simulink model "six_plus_six_AcmsteeringV10_main"  (R2014a)
settings: Solver=FixedStepDiscrete  StartTime=0.0  StopTime=10.0  FixedStep=0.0005  RelTol=1e-3
InitFcn:
  | Veh_Par_wxt
values from neighbouring files (symbols this model uses):
  acc_spdctl = [0 100]    [Veh_Par_wxt.m]
  ag_thr = ecucoder_cal(ag_thr)    [Veh_Par_wxt.m]
  B = 1.8    [Veh_Par_wxt.m]
  bra_em = 100    [Veh_Par_wxt.m]
  bra_pre_gz2 = 100/3    (= 33.3333333333)    [Veh_Par_wxt.m]
  bra_pre_gz34 = 10/3    (= 3.33333333333)    [Veh_Par_wxt.m]
  bra_pre_yd = 10/2    (= 5)    [Veh_Par_wxt.m]
  brakepre_dem_data = [0 1 2 3 4 5 6 7 8 9 10]    [Veh_Par_wxt.m]
  brakeTrq_dem_data = [0 125 251 376 502 627 753 878 1004 1129 1255]    [Veh_Par_wxt.m]
  bratrq_max = 4*1255    (= 5020)    [Veh_Par_wxt.m]
  eff_tran = 0.9    [Veh_Par_wxt.m]
  ESP_switch = ecucoder_cal(ESP_switch)    [Veh_Par_wxt.m]
  G = Mass*g    (= 15696)    [Veh_Par_wxt.m]
  kd1 = ecucoder_cal(kd1)    [Veh_Par_wxt.m]
  kd2 = 0    [Veh_Par_wxt.m]
  ki1 = ecucoder_cal(ki1)    [Veh_Par_wxt.m]
  ki2 = 1    [Veh_Par_wxt.m]
  kp1 = ecucoder_cal(kp1)    [Veh_Par_wxt.m]
  kp2 = 300    [Veh_Par_wxt.m]
  L = L1+L2    (= 2.9)    [Veh_Par_wxt.m]
  premax = 100    [Veh_Par_wxt.m]
  Radius = 0.4572/2    (= 0.2286)    [Veh_Par_wxt.m]
  RC_switch = ecucoder_cal(RC_switch)    [Veh_Par_wxt.m]
  s_opt_yi = 0.15    [Veh_Par_wxt.m]
  s_opt_zhuan = 0.8    [Veh_Par_wxt.m]
  s_opt_zhuan_add = 0.05    [Veh_Par_wxt.m]
  s_opt_zhuan_table = [0.8 0.8 0.3 0.3]    [Veh_Par_wxt.m]
  spd_map_mot = [0 499.85 999.79 1500 2000 2500 3000 3500 4000 4500 4999.8 5999.8]    [Veh_Par_wxt.m]
  spd_spdctl = [0 500]    [Veh_Par_wxt.m]
  speed_thr_park = 5/3.6/Radius*tras_ratio*30/pi    (= 464.143899364)    [Veh_Par_wxt.m]
  TCS_switch = ecucoder_cal(TCS_switch)    [Veh_Par_wxt.m]
  tras_ratio = 8    [Veh_Par_wxt.m]
  trq_map_mot = [70.5 70.012 71.154 65.797 53.917 45.159 38.073 32.685 27.48 17.133 14.949 10.07]    [Veh_Par_wxt.m]
  trqmax_yd = 70.5    [Veh_Par_wxt.m]
  trqmax_zx = 70.5    [Veh_Par_wxt.m]
  trqmaxneg = -70.5    [Veh_Par_wxt.m]
  v_gain = 0.9    [Veh_Par_wxt.m]
  v_table = [0 5 20 100]    [Veh_Par_wxt.m]
  v_thr_park = 5    [Veh_Par_wxt.m]
  zhidong_bianmazhi = [-140000 750000]    [Veh_Par_wxt.m]
  zhidong_down = -140000    [Veh_Par_wxt.m]
  zhidong_up = 750000    [Veh_Par_wxt.m]
  zhidong_youmen = [0 100]    [Veh_Par_wxt.m]
  zhuanxiang_bianmazhi = [-400000 0 400000]    [Veh_Par_wxt.m]
  zhuanxiang_down = -400000    [Veh_Par_wxt.m]
  zhuanxiang_up = 400000    [Veh_Par_wxt.m]
  zhuanxiang_youmen = [-100 0 100]    [Veh_Par_wxt.m]
undefined symbols (not defined in the file or in its folder): ecucoder_acal, guzhang_lf, guzhang_lm, guzhang_lr, guzhang_rf, guzhang_rm, guzhang_rr, myFIS
libraries: simulink x979, ec5744lib x59, fuzblock x2
(part 5 of 27)

== system six_plus_six_AcmsteeringV10_main/Data_input/2/Enabled Subsystem ==
  In2 : Inport
  Enable : EnablePort
  Add : Sum
  Constant : Constant  Value=256
  Constant1 : Constant  SampleTime=-1
  Constant3 : Constant  Value=256
  Data Type Conversion{8..13} (6 alike) : DataTypeConversion  OutDataTypeStr=uint8
  Demux1 : Demux  Outputs=6
  MATLAB Function1 : MATLAB Function  TreatAsAtomicUnit=on
  MATLAB Function3 : MATLAB Function  TreatAsAtomicUnit=on
  Memory : Memory  InheritSampleTime=on
  Product : Product
  Product2 : Product
  Saturation : Saturate  UpperLimit=5  LowerLimit=0
  Sum : Sum  Inputs=|++
  Sum1 : Sum  Inputs=|++
  Terminator1 : Terminator
  Terminator2 : Terminator
  motec_spd_4 : Outport
  motec_current_4 : Outport  Port=2
  enable_count1 : Outport  Port=3
  wires:
  MATLAB Function1/1(current_out) -> motec_current_4/1
  MATLAB Function3/1(speed_out) -> motec_spd_4/1
  Sum1/1 -> MATLAB Function1/1(current_in)
  Data Type Conversion13/1 -> Sum1/1
  Product2/1 -> Sum1/2
  Constant3/1 -> Product2/1
  Data Type Conversion12/1 -> Product2/2
  Sum/1 -> MATLAB Function3/1(speed)
  Product/1 -> Sum/2
  Constant/1 -> Product/1
  Data Type Conversion11/1 -> Product/2
  Data Type Conversion10/1 -> Sum/1
  Data Type Conversion9/1 -> Terminator2/1
  Data Type Conversion8/1 -> Terminator1/1
  Demux1/6 -> Data Type Conversion12/1
  Demux1/5 -> Data Type Conversion13/1
  Demux1/4 -> Data Type Conversion11/1
  Demux1/3 -> Data Type Conversion10/1
  Demux1/2 -> Data Type Conversion9/1
  Demux1/1 -> Data Type Conversion8/1
  In2/1 -> Demux1/1
  Constant1/1 -> Add/1
  Memory/1 -> Add/2
  Add/1 -> Saturation/1
  Saturation/1 -> enable_count1/1, Memory/1

== system six_plus_six_AcmsteeringV10_main/Data_input/3/Enabled Subsystem ==
  In2 : Inport
  Enable : EnablePort
  Add : Sum
  Constant : Constant  Value=256
  Constant1 : Constant  SampleTime=-1
  Constant3 : Constant  Value=256
  Data Type Conversion{8..13} (6 alike) : DataTypeConversion  OutDataTypeStr=uint8
  Demux1 : Demux  Outputs=6
  MATLAB Function1 : MATLAB Function  TreatAsAtomicUnit=on
  MATLAB Function3 : MATLAB Function  TreatAsAtomicUnit=on
  Memory : Memory  InheritSampleTime=on
  Product : Product
  Product2 : Product
  Saturation : Saturate  UpperLimit=5  LowerLimit=0
  Sum : Sum  Inputs=|++
  Sum1 : Sum  Inputs=|++
  Terminator1 : Terminator
  Terminator2 : Terminator
  motec_spd_3 : Outport
  motec_current_3 : Outport  Port=2
  enable_count1 : Outport  Port=3
  wires:
  MATLAB Function1/1(current_out) -> motec_current_3/1
  MATLAB Function3/1(speed_out) -> motec_spd_3/1
  Sum1/1 -> MATLAB Function1/1(current_in)
  Data Type Conversion13/1 -> Sum1/1
  Product2/1 -> Sum1/2
  Constant3/1 -> Product2/1
  Data Type Conversion12/1 -> Product2/2
  Sum/1 -> MATLAB Function3/1(speed)
  Product/1 -> Sum/2
  Constant/1 -> Product/1
  Data Type Conversion11/1 -> Product/2
  Data Type Conversion10/1 -> Sum/1
  Data Type Conversion9/1 -> Terminator2/1
  Data Type Conversion8/1 -> Terminator1/1
  Demux1/6 -> Data Type Conversion12/1
  Demux1/5 -> Data Type Conversion13/1
  Demux1/4 -> Data Type Conversion11/1
  Demux1/3 -> Data Type Conversion10/1
  Demux1/2 -> Data Type Conversion9/1
  Demux1/1 -> Data Type Conversion8/1
  In2/1 -> Demux1/1
  Constant1/1 -> Add/1
  Memory/1 -> Add/2
  Add/1 -> Saturation/1
  Saturation/1 -> enable_count1/1, Memory/1

== system six_plus_six_AcmsteeringV10_main/Data_input/4/Enabled Subsystem ==
  In2 : Inport
  Enable : EnablePort
  Data Type Conversion{,1..7} (8 alike) : DataTypeConversion
  Demux1 : Demux  Outputs=8
  MATLAB Function : MATLAB Function  TreatAsAtomicUnit=on
  MATLAB Function1 : MATLAB Function  TreatAsAtomicUnit=on
  Xangularrate_Out : Outport
  Yangularrate_Out : Outport  Port=2
  wires:
  In2/1 -> Demux1/1
  Demux1/4 -> Data Type Conversion3/1
  Demux1/3 -> Data Type Conversion2/1
  Demux1/2 -> Data Type Conversion1/1
  Demux1/1 -> Data Type Conversion/1
  MATLAB Function/1(y) -> Xangularrate_Out/1
  MATLAB Function1/1(y) -> Yangularrate_Out/1
  Demux1/5 -> Data Type Conversion4/1
  Demux1/6 -> Data Type Conversion5/1
  Demux1/7 -> Data Type Conversion6/1
  Demux1/8 -> Data Type Conversion7/1
  Data Type Conversion/1 -> MATLAB Function/1(data1)
  Data Type Conversion1/1 -> MATLAB Function/2(data2)
  Data Type Conversion2/1 -> MATLAB Function/3(data3)
  Data Type Conversion3/1 -> MATLAB Function/4(data4)
  Data Type Conversion4/1 -> MATLAB Function1/1(data1)
  Data Type Conversion5/1 -> MATLAB Function1/2(data2)
  Data Type Conversion6/1 -> MATLAB Function1/3(data3)
  Data Type Conversion7/1 -> MATLAB Function1/4(data4)

== matlab function six_plus_six_AcmsteeringV10_main/MainControl/mode_control/center_steer/center_steer/容错控制/MATLAB Function ==
  data: trq_dem_l input; trq_dem_lf output; trq_dem_lm output; trq_dem_r input; trqlim_lf input; trqlim_lm input; trqlim_lr input; trqlim_rf input; trqlim_rm input; trqlim_rr input; guzhang_lf input; guzhang_lm input; guzhang_lr input; guzhang_rf input; guzhang_rm input; guzhang_rr input; trq_dem_lr output; trq_dem_rf output; trq_dem_rm output; trq_dem_rr output; bra_pre_l output; bra_pre_r output; bra_pre_yd input; mode output; bra_dem_l input; bra_dem_r input; brake_dem input
function [trq_dem_lf,trq_dem_lm,trq_dem_lr,trq_dem_rf,trq_dem_rm,trq_dem_rr,bra_pre_l,bra_pre_r,mode] = fcn(trq_dem_l,trq_dem_r,trqlim_lf,trqlim_lm,trqlim_lr,trqlim_rf,trqlim_rm,trqlim_rr,guzhang_lf,guzhang_lm,guzhang_lr,guzhang_rf,guzhang_rm,guzhang_rr,bra_pre_yd,bra_dem_l,bra_dem_r,brake_dem)
%#codegen
if brake_dem==0
    
    trq_dem_lf=single(trq_dem_l/3);
    trq_dem_lm=single(trq_dem_l/3);
    trq_dem_lr=single(trq_dem_l/3);
    trq_dem_rf=single(trq_dem_r/3);
    trq_dem_rm=single(trq_dem_r/3);
    trq_dem_rr=single(trq_dem_r/3);
    bra_pre_l=single(0);
    bra_pre_r=single(0);
    mode=1;
    
    
    %     if guzhang_lf==0 && guzhang_lr==0 && guzhang_rf==0 && guzhang_rr==0    %0电机故障,平均分配
    %         trq_dem_lf=single(trq_dem_l/2);
    %         trq_dem_lr=single(trq_dem_l/2);
    %         trq_dem_rf=single(trq_dem_r/2);
    %         trq_dem_rr=single(trq_dem_r/2);
    %         bra_pre_l=single(0);
    %         bra_pre_r=single(0);
    %         mode=1;
    %     elseif  guzhang_lf==1 && guzhang_lr==0 && guzhang_rf==0 && guzhang_rr==0  %1电机故障，同侧电机进行力矩转移,跟行车不同，对侧不降扭。
    %         trq_dem_lf=single(0);
    %         trq_dem_lr=single(min(trq_dem_l,trqlim_lr));
    %         trq_dem_rf=single(trq_dem_r/2);
    %         trq_dem_rr=single(trq_dem_r/2);
    %         bra_pre_l=single(0);
    %         bra_pre_r=single(0);
    %         mode=2;
    %     elseif  guzhang_lf==0 && guzhang_lr==1 && guzhang_rf==0 && guzhang_rr==0
    %         trq_dem_lf=single(min(trq_dem_l,trqlim_lf));
    %         trq_dem_lr=single(0);
    %         trq_dem_rf=single(trq_dem_r/2);
    %         trq_dem_rr=single(trq_dem_r/2);
    %         bra_pre_l=single(0);
    %         bra_pre_r=single(0);
    %         mode=3;
    %     elseif  guzhang_lf==0 && guzhang_lr==0 && guzhang_rf==1 && guzhang_rr==0
    %         trq_dem_rf=single(0);
    %         trq_dem_rr=single(min(trq_dem_r,trqlim_rr));
    %         trq_dem_lf=single(trq_dem_l/2);
    %         trq_dem_lr=single(trq_dem_l/2);
    %         bra_pre_l=single(0);
    %         bra_pre_r=single(0);
    %         mode=4;
    %     elseif  guzhang_lf==0 && guzhang_lr==0 && guzhang_rf==0 && guzhang_rr==1
    %         trq_dem_rf=single(min(trq_dem_r,trqlim_rf));
    %         trq_dem_rr=single(0);
    %         trq_dem_lf=single(trq_dem_l/2);
    %         trq_dem_lr=single(trq_dem_l/2);
    %         bra_pre_l=single(0);
    %         bra_pre_r=single(0);
    %         mode=5;
    %     elseif  guzhang_lf==1 && guzhang_lr==1 && guzhang_rf==0 && guzhang_rr==0  %2电机故障，左侧双电机故障，左侧履带施加制动，改为原地转向
    %         trq_dem_lf=single(0);
    %         trq_dem_lr=single(0);
    %         trq_dem_rf=single(trq_dem_r/2);
    %         trq_dem_rr=single(trq_dem_r/2);
    %         bra_pre_l=single(bra_pre_yd);
    %         bra_pre_r=single(0);
    %         mode=6;
    %     elseif  guzhang_lf==0 && guzhang_lr==0 && guzhang_rf==1 && guzhang_rr==1  %右侧双电机故障
    %         trq_dem_lf=single(trq_dem_l/2);
    %         trq_dem_lr=single(trq_dem_l/2);
    %         trq_dem_rf=single(0);
    %         trq_dem_rr=single(0);
    %         bra_pre_l=single(0);
    %         bra_pre_r=single(bra_pre_yd);
    %         mode=7;
    %     elseif  guzhang_lf==1 && guzhang_lr==0 && guzhang_rf==1 && guzhang_rr==0 %2电机故障，对侧双电机故障,有4种情况,前两电机故障
    %         trq_dem_lf=single(0);
    %         trq_dem_rf=single(0);
    %         trq_dem_lr=single(min(trq_dem_l,trqlim_lr));
    %         trq_dem_rr=single(min(trq_dem_r,trqlim_rr));
    %         bra_pre_l=single(0);
    %         bra_pre_r=single(0);
    %         mode=8;
    %     elseif  guzhang_lf==0 && guzhang_lr==1 && guzhang_rf==0 && guzhang_rr==1 %后两电机故障
    %         trq_dem_lr=single(0);
    %         trq_dem_rr=single(0);
    %         trq_dem_lf=single(min(trq_dem_l,trqlim_lf));
    %         trq_dem_rf=single(min(trq_dem_r,trqlim_rf));
    %         bra_pre_l=single(0);
    %         bra_pre_r=single(0);
    %         mode=9;
    %     elseif  guzhang_lf==1 && guzhang_lr==0 && guzhang_rf==0 && guzhang_rr==1 %左前电机和右后电机故障
    %         trq_dem_lf=single(0);
    %         trq_dem_rr=single(0);
    %         trq_dem_lr=single(min(trq_dem_l,trqlim_lr));
    %         trq_dem_rf=single(min(trq_dem_r,trqlim_rf));
    %         bra_pre_l=single(0);
    %         bra_pre_r=single(0);
    %         mode=10;
    %     elseif  guzhang_lf==0 && guzhang_lr==1 && guzhang_rf==1 && guzhang_rr==0 %左后电机和右前电机故障
    %         trq_dem_lr=single(0);
    %         trq_dem_rf=single(0);
    %         trq_dem_lf=single(min(trq_dem_l,trqlim_lf));
    %         trq_dem_rr=single(min(trq_dem_r,trqlim_rr));
    %         bra_pre_l=single(0);
    %         bra_pre_r=single(0);
    %         mode=11;
    %     elseif guzhang_lf==1 && guzhang_lr==1 && guzhang_rf==1 && guzhang_rr==0   % 三电机故障
    %         trq_dem_lf=single(0);
    %         trq_dem_lr=single(0);
    %         trq_dem_rf=single(0);
    %         trq_dem_rr=single(min(trq_dem_r,trqlim_rr));
    %         bra_pre_l=single(bra_pre_yd);
    %         bra_pre_r=single(0);
    %         mode=12;
    %     elseif guzhang_lf==1 && guzhang_lr==1 && guzhang_rf==0 && guzhang_rr==1
    %         trq_dem_lf=single(0);
    %         trq_dem_lr=single(0);
    %         trq_dem_rf=single(min(trq_dem_r,trqlim_rf));
    %         trq_dem_rr=single(0);
    %         bra_pre_l=single(bra_pre_yd);
    %         bra_pre_r=single(0);
    %         mode=13;
    %     elseif guzhang_lf==1 && guzhang_lr==0 && guzhang_rf==1 && guzhang_rr==1
    %         trq_dem_lf=single(0);
    %         trq_dem_lr=single(min(trq_dem_l,trqlim_lr));
    %         trq_dem_rf=single(0);
    %         trq_dem_rr=single(0);
    %         bra_pre_l=single(0);
    %         bra_pre_r=single(bra_pre_yd);
    %         mode=14;
    %     elseif guzhang_lf==0 && guzhang_lr==1 && guzhang_rf==1 && guzhang_rr==1
    %         trq_dem_lf=single(min(trq_dem_l,trqlim_lf));
    %         trq_dem_lr=single(0);
    %         trq_dem_rf=single(0);
    %         trq_dem_rr=single(0);
    %         bra_pre_l=single(0);
    %         bra_pre_r=single(bra_pre_yd);
    %         mode=15;
    %     else
    %         %     guzhang_lf==1 && guzhang_lr==1 && guzhang_rf==1 && guzhang_rr==1 %四电机故障
    %         trq_dem_lf=single(0);
    %         trq_dem_lr=single(0);
    %         trq_dem_rf=single(0);
    %         trq_dem_rr=single(0);
    %         bra_pre_l=single(0);
    %         bra_pre_r=single(0);
    %         mode=16;
    %     end
else
    trq_dem_lf=single(0);
    trq_dem_lm=single(0);
    trq_dem_lr=single(0);
    trq_dem_rf=single(0);
    trq_dem_rm=single(0);
    trq_dem_rr=single(0);
    bra_pre_l=single(bra_dem_l);
    bra_pre_r=single(bra_dem_r);
    mode=17;
end
trq_dem_lf=single(min(trqlim_lf,trq_dem_lf));trq_dem_lf=single(max(0,trq_dem_lf));
trq_dem_lm=single(min(trqlim_lm,trq_dem_lm));trq_dem_lm=single(max(0,trq_dem_lm));
trq_dem_lr=single(min(trqlim_lr,trq_dem_lr));trq_dem_lr=single(max(0,trq_dem_lr));
trq_dem_rf=single(min(trqlim_rf,trq_dem_rf));trq_dem_rf=single(max(0,trq_dem_rf));
trq_dem_rm=single(min(trqlim_rm,trq_dem_rm));trq_dem_rm=single(max(0,trq_dem_rm));
trq_dem_rr=single(min(trqlim_rr,trq_dem_rr));trq_dem_rr=single(max(0,trq_dem_rr));
bra_pre_l=single(bra_pre_l);
bra_pre_r=single(bra_pre_r);
end

== system six_plus_six_AcmsteeringV10_main/Data_input/5/Enabled Subsystem ==
  In2 : Inport
  Enable : EnablePort
  Data Type Conversion{,1..7} (8 alike) : DataTypeConversion
  Demux1 : Demux  Outputs=8
  MATLAB Function : MATLAB Function  TreatAsAtomicUnit=on
  MATLAB Function1 : MATLAB Function  TreatAsAtomicUnit=on
  Zangularrate_Out : Outport
  Xacceleration_Out : Outport  Port=2
  wires:
  Demux1/8 -> Data Type Conversion7/1
  Demux1/7 -> Data Type Conversion6/1
  Demux1/6 -> Data Type Conversion5/1
  Demux1/5 -> Data Type Conversion4/1
  MATLAB Function1/1(y) -> Xacceleration_Out/1
  MATLAB Function/1(y) -> Zangularrate_Out/1
  Demux1/1 -> Data Type Conversion/1
  Demux1/2 -> Data Type Conversion1/1
  Demux1/3 -> Data Type Conversion2/1
  Demux1/4 -> Data Type Conversion3/1
  In2/1 -> Demux1/1
  Data Type Conversion/1 -> MATLAB Function/1(data1)
  Data Type Conversion1/1 -> MATLAB Function/2(data2)
  Data Type Conversion2/1 -> MATLAB Function/3(data3)
  Data Type Conversion3/1 -> MATLAB Function/4(data4)
  Data Type Conversion4/1 -> MATLAB Function1/1(data1)
  Data Type Conversion5/1 -> MATLAB Function1/2(data2)
  Data Type Conversion7/1 -> MATLAB Function1/4(data4)
  Data Type Conversion6/1 -> MATLAB Function1/3(data3)

== system six_plus_six_AcmsteeringV10_main/Data_input/6/Enabled Subsystem ==
  In2 : Inport
  Enable : EnablePort
  Data Type Conversion{,1..7} (8 alike) : DataTypeConversion
  Demux1 : Demux  Outputs=8
  MATLAB Function : MATLAB Function  TreatAsAtomicUnit=on
  MATLAB Function1 : MATLAB Function  TreatAsAtomicUnit=on
  Yacceleration_Out : Outport
  Zacceleration_Out : Outport  Port=2
  wires:
  In2/1 -> Demux1/1
  Demux1/4 -> Data Type Conversion3/1
  Demux1/3 -> Data Type Conversion2/1
  Demux1/2 -> Data Type Conversion1/1
  Demux1/1 -> Data Type Conversion/1
  MATLAB Function/1(y) -> Yacceleration_Out/1
  MATLAB Function1/1(y) -> Zacceleration_Out/1
  Demux1/5 -> Data Type Conversion4/1
  Demux1/6 -> Data Type Conversion5/1
  Demux1/7 -> Data Type Conversion6/1
  Demux1/8 -> Data Type Conversion7/1
  Data Type Conversion7/1 -> MATLAB Function1/4(data4)
  Data Type Conversion2/1 -> MATLAB Function/3(data3)
  Data Type Conversion/1 -> MATLAB Function/1(data1)
  Data Type Conversion1/1 -> MATLAB Function/2(data2)
  Data Type Conversion4/1 -> MATLAB Function1/1(data1)
  Data Type Conversion5/1 -> MATLAB Function1/2(data2)
  Data Type Conversion3/1 -> MATLAB Function/4(data4)
  Data Type Conversion6/1 -> MATLAB Function1/3(data3)

== system six_plus_six_AcmsteeringV10_main/Data_input/7/Enabled Subsystem ==
  In2 : Inport
  Enable : EnablePort
  Data Type Conversion{,1..7} (8 alike) : DataTypeConversion
  Demux1 : Demux  Outputs=8
  MATLAB Function : MATLAB Function  TreatAsAtomicUnit=on
  MATLAB Function1 : MATLAB Function  TreatAsAtomicUnit=on
  NorthSpd_Out : Outport
  SkySpd_Out : Outport  Port=2
  wires:
  Demux1/8 -> Data Type Conversion7/1
  Demux1/7 -> Data Type Conversion6/1
  Demux1/6 -> Data Type Conversion5/1
  Demux1/5 -> Data Type Conversion4/1
  MATLAB Function1/1(y) -> SkySpd_Out/1
  MATLAB Function/1(y) -> NorthSpd_Out/1
  Demux1/1 -> Data Type Conversion/1
  Demux1/2 -> Data Type Conversion1/1
  Demux1/3 -> Data Type Conversion2/1
  Demux1/4 -> Data Type Conversion3/1
  In2/1 -> Demux1/1
  Data Type Conversion/1 -> MATLAB Function/1(data1)
  Data Type Conversion2/1 -> MATLAB Function/3(data3)
  Data Type Conversion1/1 -> MATLAB Function/2(data2)
  Data Type Conversion6/1 -> MATLAB Function1/3(data3)
  Data Type Conversion5/1 -> MATLAB Function1/2(data2)
  Data Type Conversion4/1 -> MATLAB Function1/1(data1)
  Data Type Conversion7/1 -> MATLAB Function1/4(data4)
  Data Type Conversion3/1 -> MATLAB Function/4(data4)

== system six_plus_six_AcmsteeringV10_main/Data_input/8/Enabled Subsystem ==
  In2 : Inport
  Enable : EnablePort
  Data Type Conversion{,1..7} (8 alike) : DataTypeConversion
  Demux1 : Demux  Outputs=8
  MATLAB Function : MATLAB Function  TreatAsAtomicUnit=on
  MATLAB Function1 : MATLAB Function  TreatAsAtomicUnit=on
  EastSpd_Out : Outport
  Altitude_Out : Outport  Port=2
  wires:
  In2/1 -> Demux1/1
  Demux1/4 -> Data Type Conversion3/1
  Demux1/3 -> Data Type Conversion2/1
  Demux1/2 -> Data Type Conversion1/1
  Demux1/1 -> Data Type Conversion/1
  MATLAB Function/1(y) -> EastSpd_Out/1
  MATLAB Function1/1(y) -> Altitude_Out/1
  Demux1/5 -> Data Type Conversion4/1
  Demux1/6 -> Data Type Conversion5/1
  Demux1/7 -> Data Type Conversion6/1
  Demux1/8 -> Data Type Conversion7/1
  Data Type Conversion/1 -> MATLAB Function/1(data1)
  Data Type Conversion5/1 -> MATLAB Function1/2(data2)
  Data Type Conversion2/1 -> MATLAB Function/3(data3)
  Data Type Conversion1/1 -> MATLAB Function/2(data2)
  Data Type Conversion7/1 -> MATLAB Function1/4(data4)
  Data Type Conversion4/1 -> MATLAB Function1/1(data1)
  Data Type Conversion6/1 -> MATLAB Function1/3(data3)
  Data Type Conversion3/1 -> MATLAB Function/4(data4)

== system six_plus_six_AcmsteeringV10_main/Data_input/9/Enabled Subsystem ==
  In2 : Inport
  Enable : EnablePort
  Data Type Conversion{,1..7} (8 alike) : DataTypeConversion
  Demux1 : Demux  Outputs=8
  MATLAB Function : MATLAB Function  TreatAsAtomicUnit=on
  MATLAB Function1 : MATLAB Function  TreatAsAtomicUnit=on
  Longitude_Out : Outport
  Latitude_Out : Outport  Port=2
  wires:
  Demux1/8 -> Data Type Conversion7/1
  Demux1/7 -> Data Type Conversion6/1
  Demux1/6 -> Data Type Conversion5/1
  Demux1/5 -> Data Type Conversion4/1
  MATLAB Function1/1(y) -> Latitude_Out/1
  MATLAB Function/1(y) -> Longitude_Out/1
  Demux1/1 -> Data Type Conversion/1
  Demux1/2 -> Data Type Conversion1/1
  Demux1/3 -> Data Type Conversion2/1
  Demux1/4 -> Data Type Conversion3/1
  In2/1 -> Demux1/1
  Data Type Conversion4/1 -> MATLAB Function1/1(data1)
  Data Type Conversion2/1 -> MATLAB Function/3(data3)
  Data Type Conversion1/1 -> MATLAB Function/2(data2)
  Data Type Conversion3/1 -> MATLAB Function/4(data4)
  Data Type Conversion5/1 -> MATLAB Function1/2(data2)
  Data Type Conversion6/1 -> MATLAB Function1/3(data3)
  Data Type Conversion/1 -> MATLAB Function/1(data1)
  Data Type Conversion7/1 -> MATLAB Function1/4(data4)

== system six_plus_six_AcmsteeringV10_main/Data_input/BMS1/BMS1 ==
  input : Inport
  Enable : EnablePort
  BMS1_SOC_Ad : Sum
  BMS1_SOC_Convert : DataTypeConversion  OutDataTypeStr=uint32
  BMS1_SOC_F : Gain  Gain=0.1
  BMS1_SOC_L : simulink/Logic and Bit Operations/Bitwise Operator  logicop=AND  UseBitMask=on  BitMask=65535  BitMaskRealWorld=Stored Integer
  BMS1_SOC_O : Constant  Value=0  OutDataTypeStr=single
  BMS1_SOC_S : ArithShift
  BMS1_SOC_Sub : Subsystem
  BMS1_SOC_sat : Saturate  UpperLimit=1000  LowerLimit=0
  BMS1_SOCcv : DataTypeConversion
  BMS1_SOCinput5_Ad : Sum
  BMS1_SOCinput5_C : Constant  Value=256
  BMS1_SOCinput5_P : Product
  BMS1_Sys_Status1_Ad : Sum
  BMS1_Sys_Status1_Convert : DataTypeConversion  OutDataTypeStr=uint32
  BMS1_Sys_Status1_F : Gain
  BMS1_Sys_Status1_L : simulink/Logic and Bit Operations/Bitwise Operator  logicop=AND  UseBitMask=on  BitMask=255  BitMaskRealWorld=Stored Integer
  BMS1_Sys_Status1_O : Constant  Value=0  OutDataTypeStr=single
  BMS1_Sys_Status1_S : ArithShift
  BMS1_Sys_Status1_Sub : Subsystem
  BMS1_Sys_Status1_sat : Saturate  UpperLimit=255  LowerLimit=0
  BMS1_Sys_Status1cv : DataTypeConversion
  BMS1_Sys_Status2_Ad : Sum
  BMS1_Sys_Status2_Convert : DataTypeConversion  OutDataTypeStr=uint32
  BMS1_Sys_Status2_F : Gain
  BMS1_Sys_Status2_L : simulink/Logic and Bit Operations/Bitwise Operator  logicop=AND  UseBitMask=on  BitMask=255  BitMaskRealWorld=Stored Integer
  BMS1_Sys_Status2_O : Constant  Value=0  OutDataTypeStr=single
  BMS1_Sys_Status2_S : ArithShift
  BMS1_Sys_Status2_Sub : Subsystem
  BMS1_Sys_Status2_sat : Saturate  UpperLimit=255  LowerLimit=0
  BMS1_Sys_Status2cv : DataTypeConversion
  BMS1_TotalCurrent_Ad : Sum
  BMS1_TotalCurrent_Convert : DataTypeConversion  OutDataTypeStr=uint32
  BMS1_TotalCurrent_F : Gain  Gain=0.1
  BMS1_TotalCurrent_L : simulink/Logic and Bit Operations/Bitwise Operator  logicop=AND  UseBitMask=on  BitMask=65535  BitMaskRealWorld=Stored Integer
  BMS1_TotalCurrent_O : Constant  Value=-32000  OutDataTypeStr=single
  BMS1_TotalCurrent_S : ArithShift
  BMS1_TotalCurrent_Sub : Subsystem
  BMS1_TotalCurrent_sat : Saturate  UpperLimit=3353.5  LowerLimit=-32000
  BMS1_TotalCurrentcv : DataTypeConversion
  BMS1_TotalCurrentinput3_Ad : Sum
  BMS1_TotalCurrentinput3_C : Constant  Value=256
  BMS1_TotalCurrentinput3_P : Product
  BMS1_TotalVol_Ad : Sum
  BMS1_TotalVol_Convert : DataTypeConversion  OutDataTypeStr=uint32
  BMS1_TotalVol_F : Gain  Gain=0.1
  BMS1_TotalVol_L : simulink/Logic and Bit Operations/Bitwise Operator  logicop=AND  UseBitMask=on  BitMask=65535  BitMaskRealWorld=Stored Integer
  BMS1_TotalVol_O : Constant  Value=0  OutDataTypeStr=single
  BMS1_TotalVol_S : ArithShift
  BMS1_TotalVol_Sub : Subsystem
  BMS1_TotalVol_sat : Saturate  UpperLimit=6553.5  LowerLimit=0
  BMS1_TotalVolcv : DataTypeConversion
  BMS1_TotalVolinput1_Ad : Sum
  BMS1_TotalVolinput1_C : Constant  Value=256
  BMS1_TotalVolinput1_P : Product
  Demux : Demux  Outputs=8
  BMS1_TotalVol_Out : Outport
  BMS1_TotalCurrent_Out : Outport  Port=2
  BMS1_Sys_Status2_Out : Outport  Port=3
  BMS1_Sys_Status1_Out : Outport  Port=4
  BMS1_SOC_Out : Outport  Port=5
  wires:
  BMS1_TotalVol_F/1 -> BMS1_TotalVol_Ad/1
  BMS1_TotalVol_O/1 -> BMS1_TotalVol_Ad/2
  BMS1_TotalVol_Ad/1 -> BMS1_TotalVol_sat/1
  BMS1_TotalVol_sat/1 -> BMS1_TotalVol_Out/1
  Demux/1 -> BMS1_TotalVolinput1_P/1
  BMS1_TotalVolinput1_C/1 -> BMS1_TotalVolinput1_P/2
  BMS1_TotalVolinput1_P/1 -> BMS1_TotalVolinput1_Ad/1
  Demux/2 -> BMS1_TotalVolinput1_Ad/2
  BMS1_TotalVolinput1_Ad/1 -> BMS1_TotalVol_Sub/1(In1)
  BMS1_TotalVol_Sub/1(Out1) -> BMS1_TotalVol_Convert/1
  BMS1_TotalVol_Convert/1 -> BMS1_TotalVol_L/1
  BMS1_TotalVol_L/1 -> BMS1_TotalVol_S/1
  BMS1_TotalVol_S/1 -> BMS1_TotalVolcv/1
  BMS1_TotalVolcv/1 -> BMS1_TotalVol_F/1
  BMS1_TotalCurrent_F/1 -> BMS1_TotalCurrent_Ad/1
  BMS1_TotalCurrent_O/1 -> BMS1_TotalCurrent_Ad/2
  BMS1_TotalCurrent_Ad/1 -> BMS1_TotalCurrent_sat/1
  BMS1_TotalCurrent_sat/1 -> BMS1_TotalCurrent_Out/1
  Demux/3 -> BMS1_TotalCurrentinput3_P/1
  BMS1_TotalCurrentinput3_C/1 -> BMS1_TotalCurrentinput3_P/2
  BMS1_TotalCurrentinput3_P/1 -> BMS1_TotalCurrentinput3_Ad/1
  Demux/4 -> BMS1_TotalCurrentinput3_Ad/2
  BMS1_TotalCurrentinput3_Ad/1 -> BMS1_TotalCurrent_Sub/1(In1)
  BMS1_TotalCurrent_Sub/1(Out1) -> BMS1_TotalCurrent_Convert/1
  BMS1_TotalCurrent_Convert/1 -> BMS1_TotalCurrent_L/1
  BMS1_TotalCurrent_L/1 -> BMS1_TotalCurrent_S/1
  BMS1_TotalCurrent_S/1 -> BMS1_TotalCurrentcv/1
  BMS1_TotalCurrentcv/1 -> BMS1_TotalCurrent_F/1
  BMS1_Sys_Status2_F/1 -> BMS1_Sys_Status2_Ad/1
  BMS1_Sys_Status2_O/1 -> BMS1_Sys_Status2_Ad/2
  BMS1_Sys_Status2_Ad/1 -> BMS1_Sys_Status2_sat/1
  BMS1_Sys_Status2_sat/1 -> BMS1_Sys_Status2_Out/1
  Demux/8 -> BMS1_Sys_Status2_Sub/1(In1)
  BMS1_Sys_Status2_Sub/1(Out1) -> BMS1_Sys_Status2_Convert/1
  BMS1_Sys_Status2_Convert/1 -> BMS1_Sys_Status2_L/1
  BMS1_Sys_Status2_L/1 -> BMS1_Sys_Status2_S/1
  BMS1_Sys_Status2_S/1 -> BMS1_Sys_Status2cv/1
  BMS1_Sys_Status2cv/1 -> BMS1_Sys_Status2_F/1
  BMS1_Sys_Status1_F/1 -> BMS1_Sys_Status1_Ad/1
  BMS1_Sys_Status1_O/1 -> BMS1_Sys_Status1_Ad/2
  BMS1_Sys_Status1_Ad/1 -> BMS1_Sys_Status1_sat/1
  BMS1_Sys_Status1_sat/1 -> BMS1_Sys_Status1_Out/1
  Demux/7 -> BMS1_Sys_Status1_Sub/1(In1)
  BMS1_Sys_Status1_Sub/1(Out1) -> BMS1_Sys_Status1_Convert/1
  BMS1_Sys_Status1_Convert/1 -> BMS1_Sys_Status1_L/1
  BMS1_Sys_Status1_L/1 -> BMS1_Sys_Status1_S/1
  BMS1_Sys_Status1_S/1 -> BMS1_Sys_Status1cv/1
  BMS1_Sys_Status1cv/1 -> BMS1_Sys_Status1_F/1
  BMS1_SOC_F/1 -> BMS1_SOC_Ad/1
  BMS1_SOC_O/1 -> BMS1_SOC_Ad/2
  BMS1_SOC_Ad/1 -> BMS1_SOC_sat/1
  BMS1_SOC_sat/1 -> BMS1_SOC_Out/1
  Demux/5 -> BMS1_SOCinput5_P/1
  BMS1_SOCinput5_C/1 -> BMS1_SOCinput5_P/2
  BMS1_SOCinput5_P/1 -> BMS1_SOCinput5_Ad/1
  Demux/6 -> BMS1_SOCinput5_Ad/2
  BMS1_SOCinput5_Ad/1 -> BMS1_SOC_Sub/1(In1)
  BMS1_SOC_Sub/1(Out1) -> BMS1_SOC_Convert/1
  BMS1_SOC_Convert/1 -> BMS1_SOC_L/1
  BMS1_SOC_L/1 -> BMS1_SOC_S/1
  BMS1_SOC_S/1 -> BMS1_SOCcv/1
  BMS1_SOCcv/1 -> BMS1_SOC_F/1
  input/1 -> Demux/1

== system six_plus_six_AcmsteeringV10_main/Data_input/BMS1-2/BMS1 ==
  input : Inport
  Enable : EnablePort
  BMS1_SOC_Ad : Sum
  BMS1_SOC_Convert : DataTypeConversion  OutDataTypeStr=uint32
  BMS1_SOC_F : Gain  Gain=0.1
  BMS1_SOC_L : simulink/Logic and Bit Operations/Bitwise Operator  logicop=AND  UseBitMask=on  BitMask=65535  BitMaskRealWorld=Stored Integer
  BMS1_SOC_O : Constant  Value=0  OutDataTypeStr=single
  BMS1_SOC_S : ArithShift
  BMS1_SOC_Sub : Subsystem
  BMS1_SOC_sat : Saturate  UpperLimit=1000  LowerLimit=0
  BMS1_SOCcv : DataTypeConversion
  BMS1_SOCinput5_Ad : Sum
  BMS1_SOCinput5_C : Constant  Value=256
  BMS1_SOCinput5_P : Product
  BMS1_Sys_Status1_Ad : Sum
  BMS1_Sys_Status1_Convert : DataTypeConversion  OutDataTypeStr=uint32
  BMS1_Sys_Status1_F : Gain
  BMS1_Sys_Status1_L : simulink/Logic and Bit Operations/Bitwise Operator  logicop=AND  UseBitMask=on  BitMask=255  BitMaskRealWorld=Stored Integer
  BMS1_Sys_Status1_O : Constant  Value=0  OutDataTypeStr=single
  BMS1_Sys_Status1_S : ArithShift
  BMS1_Sys_Status1_Sub : Subsystem
  BMS1_Sys_Status1_sat : Saturate  UpperLimit=255  LowerLimit=0
  BMS1_Sys_Status1cv : DataTypeConversion
  BMS1_Sys_Status2_Ad : Sum
  BMS1_Sys_Status2_Convert : DataTypeConversion  OutDataTypeStr=uint32
  BMS1_Sys_Status2_F : Gain
  BMS1_Sys_Status2_L : simulink/Logic and Bit Operations/Bitwise Operator  logicop=AND  UseBitMask=on  BitMask=255  BitMaskRealWorld=Stored Integer
  BMS1_Sys_Status2_O : Constant  Value=0  OutDataTypeStr=single
  BMS1_Sys_Status2_S : ArithShift
  BMS1_Sys_Status2_Sub : Subsystem
  BMS1_Sys_Status2_sat : Saturate  UpperLimit=255  LowerLimit=0
  BMS1_Sys_Status2cv : DataTypeConversion
  BMS1_TotalCurrent_Ad : Sum
  BMS1_TotalCurrent_Convert : DataTypeConversion  OutDataTypeStr=uint32
  BMS1_TotalCurrent_F : Gain  Gain=0.1
  BMS1_TotalCurrent_L : simulink/Logic and Bit Operations/Bitwise Operator  logicop=AND  UseBitMask=on  BitMask=65535  BitMaskRealWorld=Stored Integer
  BMS1_TotalCurrent_O : Constant  Value=-32000  OutDataTypeStr=single
  BMS1_TotalCurrent_S : ArithShift
  BMS1_TotalCurrent_Sub : Subsystem
  BMS1_TotalCurrent_sat : Saturate  UpperLimit=3353.5  LowerLimit=-32000
  BMS1_TotalCurrentcv : DataTypeConversion
  BMS1_TotalCurrentinput3_Ad : Sum
  BMS1_TotalCurrentinput3_C : Constant  Value=256
  BMS1_TotalCurrentinput3_P : Product
  BMS1_TotalVol_Ad : Sum
  BMS1_TotalVol_Convert : DataTypeConversion  OutDataTypeStr=uint32
  BMS1_TotalVol_F : Gain  Gain=0.1
  BMS1_TotalVol_L : simulink/Logic and Bit Operations/Bitwise Operator  logicop=AND  UseBitMask=on  BitMask=65535  BitMaskRealWorld=Stored Integer
  BMS1_TotalVol_O : Constant  Value=0  OutDataTypeStr=single
  BMS1_TotalVol_S : ArithShift
  BMS1_TotalVol_Sub : Subsystem
  BMS1_TotalVol_sat : Saturate  UpperLimit=6553.5  LowerLimit=0
  BMS1_TotalVolcv : DataTypeConversion
  BMS1_TotalVolinput1_Ad : Sum
  BMS1_TotalVolinput1_C : Constant  Value=256
  BMS1_TotalVolinput1_P : Product
  Demux : Demux  Outputs=8
  BMS1_TotalVol_Out : Outport
  BMS1_TotalCurrent_Out : Outport  Port=2
  BMS1_Sys_Status2_Out : Outport  Port=3
  BMS1_Sys_Status1_Out : Outport  Port=4
  BMS1_SOC_Out : Outport  Port=5
  wires:
  BMS1_TotalVol_F/1 -> BMS1_TotalVol_Ad/1
  BMS1_TotalVol_O/1 -> BMS1_TotalVol_Ad/2
  BMS1_TotalVol_Ad/1 -> BMS1_TotalVol_sat/1
  BMS1_TotalVol_sat/1 -> BMS1_TotalVol_Out/1
  Demux/1 -> BMS1_TotalVolinput1_P/1
  BMS1_TotalVolinput1_C/1 -> BMS1_TotalVolinput1_P/2
  BMS1_TotalVolinput1_P/1 -> BMS1_TotalVolinput1_Ad/1
  Demux/2 -> BMS1_TotalVolinput1_Ad/2
  BMS1_TotalVolinput1_Ad/1 -> BMS1_TotalVol_Sub/1(In1)
  BMS1_TotalVol_Sub/1(Out1) -> BMS1_TotalVol_Convert/1
  BMS1_TotalVol_Convert/1 -> BMS1_TotalVol_L/1
  BMS1_TotalVol_L/1 -> BMS1_TotalVol_S/1
  BMS1_TotalVol_S/1 -> BMS1_TotalVolcv/1
  BMS1_TotalVolcv/1 -> BMS1_TotalVol_F/1
  BMS1_TotalCurrent_F/1 -> BMS1_TotalCurrent_Ad/1
  BMS1_TotalCurrent_O/1 -> BMS1_TotalCurrent_Ad/2
  BMS1_TotalCurrent_Ad/1 -> BMS1_TotalCurrent_sat/1
  BMS1_TotalCurrent_sat/1 -> BMS1_TotalCurrent_Out/1
  Demux/3 -> BMS1_TotalCurrentinput3_P/1
  BMS1_TotalCurrentinput3_C/1 -> BMS1_TotalCurrentinput3_P/2
  BMS1_TotalCurrentinput3_P/1 -> BMS1_TotalCurrentinput3_Ad/1
  Demux/4 -> BMS1_TotalCurrentinput3_Ad/2
  BMS1_TotalCurrentinput3_Ad/1 -> BMS1_TotalCurrent_Sub/1(In1)
  BMS1_TotalCurrent_Sub/1(Out1) -> BMS1_TotalCurrent_Convert/1
  BMS1_TotalCurrent_Convert/1 -> BMS1_TotalCurrent_L/1
  BMS1_TotalCurrent_L/1 -> BMS1_TotalCurrent_S/1
  BMS1_TotalCurrent_S/1 -> BMS1_TotalCurrentcv/1
  BMS1_TotalCurrentcv/1 -> BMS1_TotalCurrent_F/1
  BMS1_Sys_Status2_F/1 -> BMS1_Sys_Status2_Ad/1
  BMS1_Sys_Status2_O/1 -> BMS1_Sys_Status2_Ad/2
  BMS1_Sys_Status2_Ad/1 -> BMS1_Sys_Status2_sat/1
  BMS1_Sys_Status2_sat/1 -> BMS1_Sys_Status2_Out/1
  Demux/8 -> BMS1_Sys_Status2_Sub/1(In1)
  BMS1_Sys_Status2_Sub/1(Out1) -> BMS1_Sys_Status2_Convert/1
  BMS1_Sys_Status2_Convert/1 -> BMS1_Sys_Status2_L/1
  BMS1_Sys_Status2_L/1 -> BMS1_Sys_Status2_S/1
  BMS1_Sys_Status2_S/1 -> BMS1_Sys_Status2cv/1
  BMS1_Sys_Status2cv/1 -> BMS1_Sys_Status2_F/1
  BMS1_Sys_Status1_F/1 -> BMS1_Sys_Status1_Ad/1
  BMS1_Sys_Status1_O/1 -> BMS1_Sys_Status1_Ad/2
  BMS1_Sys_Status1_Ad/1 -> BMS1_Sys_Status1_sat/1
  BMS1_Sys_Status1_sat/1 -> BMS1_Sys_Status1_Out/1
  Demux/7 -> BMS1_Sys_Status1_Sub/1(In1)
  BMS1_Sys_Status1_Sub/1(Out1) -> BMS1_Sys_Status1_Convert/1
  BMS1_Sys_Status1_Convert/1 -> BMS1_Sys_Status1_L/1
  BMS1_Sys_Status1_L/1 -> BMS1_Sys_Status1_S/1
  BMS1_Sys_Status1_S/1 -> BMS1_Sys_Status1cv/1
  BMS1_Sys_Status1cv/1 -> BMS1_Sys_Status1_F/1
  BMS1_SOC_F/1 -> BMS1_SOC_Ad/1
  BMS1_SOC_O/1 -> BMS1_SOC_Ad/2
  BMS1_SOC_Ad/1 -> BMS1_SOC_sat/1
  BMS1_SOC_sat/1 -> BMS1_SOC_Out/1
  Demux/5 -> BMS1_SOCinput5_P/1
  BMS1_SOCinput5_C/1 -> BMS1_SOCinput5_P/2
  BMS1_SOCinput5_P/1 -> BMS1_SOCinput5_Ad/1
  Demux/6 -> BMS1_SOCinput5_Ad/2
  BMS1_SOCinput5_Ad/1 -> BMS1_SOC_Sub/1(In1)
  BMS1_SOC_Sub/1(Out1) -> BMS1_SOC_Convert/1
  BMS1_SOC_Convert/1 -> BMS1_SOC_L/1
  BMS1_SOC_L/1 -> BMS1_SOC_S/1
  BMS1_SOC_S/1 -> BMS1_SOCcv/1
  BMS1_SOCcv/1 -> BMS1_SOC_F/1
  input/1 -> Demux/1

== system six_plus_six_AcmsteeringV10_main/Data_input/BMS1_1/BMS1 ==
  input : Inport
  Enable : EnablePort
  BMS1_SOC_Ad : Sum
  BMS1_SOC_Convert : DataTypeConversion  OutDataTypeStr=uint32
  BMS1_SOC_F : Gain  Gain=0.1
  BMS1_SOC_L : simulink/Logic and Bit Operations/Bitwise Operator  logicop=AND  UseBitMask=on  BitMask=65535  BitMaskRealWorld=Stored Integer
  BMS1_SOC_O : Constant  Value=0  OutDataTypeStr=single
  BMS1_SOC_S : ArithShift
  BMS1_SOC_Sub : Subsystem
  BMS1_SOC_sat : Saturate  UpperLimit=1000  LowerLimit=0
  BMS1_SOCcv : DataTypeConversion
  BMS1_SOCinput5_Ad : Sum
  BMS1_SOCinput5_C : Constant  Value=256
  BMS1_SOCinput5_P : Product
  BMS1_Sys_Status1_Ad : Sum
  BMS1_Sys_Status1_Convert : DataTypeConversion  OutDataTypeStr=uint32
  BMS1_Sys_Status1_F : Gain
  BMS1_Sys_Status1_L : simulink/Logic and Bit Operations/Bitwise Operator  logicop=AND  UseBitMask=on  BitMask=255  BitMaskRealWorld=Stored Integer
  BMS1_Sys_Status1_O : Constant  Value=0  OutDataTypeStr=single
  BMS1_Sys_Status1_S : ArithShift
  BMS1_Sys_Status1_Sub : Subsystem
  BMS1_Sys_Status1_sat : Saturate  UpperLimit=255  LowerLimit=0
  BMS1_Sys_Status1cv : DataTypeConversion
  BMS1_Sys_Status2_Ad : Sum
  BMS1_Sys_Status2_Convert : DataTypeConversion  OutDataTypeStr=uint32
  BMS1_Sys_Status2_F : Gain
  BMS1_Sys_Status2_L : simulink/Logic and Bit Operations/Bitwise Operator  logicop=AND  UseBitMask=on  BitMask=255  BitMaskRealWorld=Stored Integer
  BMS1_Sys_Status2_O : Constant  Value=0  OutDataTypeStr=single
  BMS1_Sys_Status2_S : ArithShift
  BMS1_Sys_Status2_Sub : Subsystem
  BMS1_Sys_Status2_sat : Saturate  UpperLimit=255  LowerLimit=0
  BMS1_Sys_Status2cv : DataTypeConversion
  BMS1_TotalCurrent_Ad : Sum
  BMS1_TotalCurrent_Convert : DataTypeConversion  OutDataTypeStr=uint32
  BMS1_TotalCurrent_F : Gain  Gain=0.1
  BMS1_TotalCurrent_L : simulink/Logic and Bit Operations/Bitwise Operator  logicop=AND  UseBitMask=on  BitMask=65535  BitMaskRealWorld=Stored Integer
  BMS1_TotalCurrent_O : Constant  Value=-32000  OutDataTypeStr=single
  BMS1_TotalCurrent_S : ArithShift
  BMS1_TotalCurrent_Sub : Subsystem
  BMS1_TotalCurrent_sat : Saturate  UpperLimit=3353.5  LowerLimit=-32000
  BMS1_TotalCurrentcv : DataTypeConversion
  BMS1_TotalCurrentinput3_Ad : Sum
  BMS1_TotalCurrentinput3_C : Constant  Value=256
  BMS1_TotalCurrentinput3_P : Product
  BMS1_TotalVol_Ad : Sum
  BMS1_TotalVol_Convert : DataTypeConversion  OutDataTypeStr=uint32
  BMS1_TotalVol_F : Gain  Gain=0.1
  BMS1_TotalVol_L : simulink/Logic and Bit Operations/Bitwise Operator  logicop=AND  UseBitMask=on  BitMask=65535  BitMaskRealWorld=Stored Integer
  BMS1_TotalVol_O : Constant  Value=0  OutDataTypeStr=single
  BMS1_TotalVol_S : ArithShift
  BMS1_TotalVol_Sub : Subsystem
  BMS1_TotalVol_sat : Saturate  UpperLimit=6553.5  LowerLimit=0
  BMS1_TotalVolcv : DataTypeConversion
  BMS1_TotalVolinput1_Ad : Sum
  BMS1_TotalVolinput1_C : Constant  Value=256
  BMS1_TotalVolinput1_P : Product
  Demux : Demux  Outputs=8
  BMS1_TotalVol_Out : Outport
  BMS1_TotalCurrent_Out : Outport  Port=2
  BMS1_Sys_Status2_Out : Outport  Port=3
  BMS1_Sys_Status1_Out : Outport  Port=4
  BMS1_SOC_Out : Outport  Port=5
  wires:
  BMS1_TotalVol_F/1 -> BMS1_TotalVol_Ad/1
  BMS1_TotalVol_O/1 -> BMS1_TotalVol_Ad/2
  BMS1_TotalVol_Ad/1 -> BMS1_TotalVol_sat/1
  BMS1_TotalVol_sat/1 -> BMS1_TotalVol_Out/1
  Demux/1 -> BMS1_TotalVolinput1_P/1
  BMS1_TotalVolinput1_C/1 -> BMS1_TotalVolinput1_P/2
  BMS1_TotalVolinput1_P/1 -> BMS1_TotalVolinput1_Ad/1
  Demux/2 -> BMS1_TotalVolinput1_Ad/2
  BMS1_TotalVolinput1_Ad/1 -> BMS1_TotalVol_Sub/1(In1)
  BMS1_TotalVol_Sub/1(Out1) -> BMS1_TotalVol_Convert/1
  BMS1_TotalVol_Convert/1 -> BMS1_TotalVol_L/1
  BMS1_TotalVol_L/1 -> BMS1_TotalVol_S/1
  BMS1_TotalVol_S/1 -> BMS1_TotalVolcv/1
  BMS1_TotalVolcv/1 -> BMS1_TotalVol_F/1
  BMS1_TotalCurrent_F/1 -> BMS1_TotalCurrent_Ad/1
  BMS1_TotalCurrent_O/1 -> BMS1_TotalCurrent_Ad/2
  BMS1_TotalCurrent_Ad/1 -> BMS1_TotalCurrent_sat/1
  BMS1_TotalCurrent_sat/1 -> BMS1_TotalCurrent_Out/1
  Demux/3 -> BMS1_TotalCurrentinput3_P/1
  BMS1_TotalCurrentinput3_C/1 -> BMS1_TotalCurrentinput3_P/2
  BMS1_TotalCurrentinput3_P/1 -> BMS1_TotalCurrentinput3_Ad/1
  Demux/4 -> BMS1_TotalCurrentinput3_Ad/2
  BMS1_TotalCurrentinput3_Ad/1 -> BMS1_TotalCurrent_Sub/1(In1)
  BMS1_TotalCurrent_Sub/1(Out1) -> BMS1_TotalCurrent_Convert/1
  BMS1_TotalCurrent_Convert/1 -> BMS1_TotalCurrent_L/1
  BMS1_TotalCurrent_L/1 -> BMS1_TotalCurrent_S/1
  BMS1_TotalCurrent_S/1 -> BMS1_TotalCurrentcv/1
  BMS1_TotalCurrentcv/1 -> BMS1_TotalCurrent_F/1
  BMS1_Sys_Status2_F/1 -> BMS1_Sys_Status2_Ad/1
  BMS1_Sys_Status2_O/1 -> BMS1_Sys_Status2_Ad/2
  BMS1_Sys_Status2_Ad/1 -> BMS1_Sys_Status2_sat/1
  BMS1_Sys_Status2_sat/1 -> BMS1_Sys_Status2_Out/1
  Demux/8 -> BMS1_Sys_Status2_Sub/1(In1)
  BMS1_Sys_Status2_Sub/1(Out1) -> BMS1_Sys_Status2_Convert/1
  BMS1_Sys_Status2_Convert/1 -> BMS1_Sys_Status2_L/1
  BMS1_Sys_Status2_L/1 -> BMS1_Sys_Status2_S/1
  BMS1_Sys_Status2_S/1 -> BMS1_Sys_Status2cv/1
  BMS1_Sys_Status2cv/1 -> BMS1_Sys_Status2_F/1
  BMS1_Sys_Status1_F/1 -> BMS1_Sys_Status1_Ad/1
  BMS1_Sys_Status1_O/1 -> BMS1_Sys_Status1_Ad/2
  BMS1_Sys_Status1_Ad/1 -> BMS1_Sys_Status1_sat/1
  BMS1_Sys_Status1_sat/1 -> BMS1_Sys_Status1_Out/1
  Demux/7 -> BMS1_Sys_Status1_Sub/1(In1)
  BMS1_Sys_Status1_Sub/1(Out1) -> BMS1_Sys_Status1_Convert/1
  BMS1_Sys_Status1_Convert/1 -> BMS1_Sys_Status1_L/1
  BMS1_Sys_Status1_L/1 -> BMS1_Sys_Status1_S/1
  BMS1_Sys_Status1_S/1 -> BMS1_Sys_Status1cv/1
  BMS1_Sys_Status1cv/1 -> BMS1_Sys_Status1_F/1
  BMS1_SOC_F/1 -> BMS1_SOC_Ad/1
  BMS1_SOC_O/1 -> BMS1_SOC_Ad/2
  BMS1_SOC_Ad/1 -> BMS1_SOC_sat/1
  BMS1_SOC_sat/1 -> BMS1_SOC_Out/1
  Demux/5 -> BMS1_SOCinput5_P/1
  BMS1_SOCinput5_C/1 -> BMS1_SOCinput5_P/2
  BMS1_SOCinput5_P/1 -> BMS1_SOCinput5_Ad/1
  Demux/6 -> BMS1_SOCinput5_Ad/2
  BMS1_SOCinput5_Ad/1 -> BMS1_SOC_Sub/1(In1)
  BMS1_SOC_Sub/1(Out1) -> BMS1_SOC_Convert/1
  BMS1_SOC_Convert/1 -> BMS1_SOC_L/1
  BMS1_SOC_L/1 -> BMS1_SOC_S/1
  BMS1_SOC_S/1 -> BMS1_SOCcv/1
  BMS1_SOCcv/1 -> BMS1_SOC_F/1
  input/1 -> Demux/1

== system six_plus_six_AcmsteeringV10_main/Data_input/BMS2/BMS2 ==
  input : Inport
  Enable : EnablePort
  BMS2_HighSingleVol_Ad : Sum
  BMS2_HighSingleVol_Convert : DataTypeConversion  OutDataTypeStr=uint32
  BMS2_HighSingleVol_F : Gain
  BMS2_HighSingleVol_L : simulink/Logic and Bit Operations/Bitwise Operator  logicop=AND  UseBitMask=on  BitMask=65535  BitMaskRealWorld=Stored Integer
  BMS2_HighSingleVol_O : Constant  Value=0  OutDataTypeStr=single
  BMS2_HighSingleVol_S : ArithShift
  BMS2_HighSingleVol_Sub : Subsystem
  BMS2_HighSingleVol_sat : Saturate  UpperLimit=10  LowerLimit=0
  BMS2_HighSingleVolcv : DataTypeConversion
  BMS2_HighSingleVolinput1_Ad : Sum
  BMS2_HighSingleVolinput1_C : Constant  Value=256
  BMS2_HighSingleVolinput1_P : Product
  BMS2_LowSingleVol_Ad : Sum
  BMS2_LowSingleVol_Convert : DataTypeConversion  OutDataTypeStr=uint32
  BMS2_LowSingleVol_F : Gain
  BMS2_LowSingleVol_L : simulink/Logic and Bit Operations/Bitwise Operator  logicop=AND  UseBitMask=on  BitMask=65535  BitMaskRealWorld=Stored Integer
  BMS2_LowSingleVol_O : Constant  Value=0  OutDataTypeStr=single
  BMS2_LowSingleVol_S : ArithShift
  BMS2_LowSingleVol_Sub : Subsystem
  BMS2_LowSingleVol_sat : Saturate  UpperLimit=65535  LowerLimit=0
  BMS2_LowSingleVolcv : DataTypeConversion
  BMS2_LowSingleVolinput3_Ad : Sum
  BMS2_LowSingleVolinput3_C : Constant  Value=256
  BMS2_LowSingleVolinput3_P : Product
  Demux : Demux  Outputs=8
  BMS2_LowSingleVol_Out : Outport
  BMS2_HighSingleVol_Out : Outport  Port=2
  wires:
  BMS2_LowSingleVol_F/1 -> BMS2_LowSingleVol_Ad/1
  BMS2_LowSingleVol_O/1 -> BMS2_LowSingleVol_Ad/2
  BMS2_LowSingleVol_Ad/1 -> BMS2_LowSingleVol_sat/1
  BMS2_LowSingleVol_sat/1 -> BMS2_LowSingleVol_Out/1
  Demux/3 -> BMS2_LowSingleVolinput3_P/1
  BMS2_LowSingleVolinput3_C/1 -> BMS2_LowSingleVolinput3_P/2
  BMS2_LowSingleVolinput3_P/1 -> BMS2_LowSingleVolinput3_Ad/1
  Demux/4 -> BMS2_LowSingleVolinput3_Ad/2
  BMS2_LowSingleVolinput3_Ad/1 -> BMS2_LowSingleVol_Sub/1(In1)
  BMS2_LowSingleVol_Sub/1(Out1) -> BMS2_LowSingleVol_Convert/1
  BMS2_LowSingleVol_Convert/1 -> BMS2_LowSingleVol_L/1
  BMS2_LowSingleVol_L/1 -> BMS2_LowSingleVol_S/1
  BMS2_LowSingleVol_S/1 -> BMS2_LowSingleVolcv/1
  BMS2_LowSingleVolcv/1 -> BMS2_LowSingleVol_F/1
  BMS2_HighSingleVol_F/1 -> BMS2_HighSingleVol_Ad/1
  BMS2_HighSingleVol_O/1 -> BMS2_HighSingleVol_Ad/2
  BMS2_HighSingleVol_Ad/1 -> BMS2_HighSingleVol_sat/1
  BMS2_HighSingleVol_sat/1 -> BMS2_HighSingleVol_Out/1
  Demux/1 -> BMS2_HighSingleVolinput1_P/1
  BMS2_HighSingleVolinput1_C/1 -> BMS2_HighSingleVolinput1_P/2
  BMS2_HighSingleVolinput1_P/1 -> BMS2_HighSingleVolinput1_Ad/1
  Demux/2 -> BMS2_HighSingleVolinput1_Ad/2
  BMS2_HighSingleVolinput1_Ad/1 -> BMS2_HighSingleVol_Sub/1(In1)
  BMS2_HighSingleVol_Sub/1(Out1) -> BMS2_HighSingleVol_Convert/1
  BMS2_HighSingleVol_Convert/1 -> BMS2_HighSingleVol_L/1
  BMS2_HighSingleVol_L/1 -> BMS2_HighSingleVol_S/1
  BMS2_HighSingleVol_S/1 -> BMS2_HighSingleVolcv/1
  BMS2_HighSingleVolcv/1 -> BMS2_HighSingleVol_F/1
  input/1 -> Demux/1

== system six_plus_six_AcmsteeringV10_main/Data_input/BMS2_1/BMS2 ==
  input : Inport
  Enable : EnablePort
  BMS2_HighSingleVol_Ad : Sum
  BMS2_HighSingleVol_Convert : DataTypeConversion  OutDataTypeStr=uint32
  BMS2_HighSingleVol_F : Gain
  BMS2_HighSingleVol_L : simulink/Logic and Bit Operations/Bitwise Operator  logicop=AND  UseBitMask=on  BitMask=65535  BitMaskRealWorld=Stored Integer
  BMS2_HighSingleVol_O : Constant  Value=0  OutDataTypeStr=single
  BMS2_HighSingleVol_S : ArithShift
  BMS2_HighSingleVol_Sub : Subsystem
  BMS2_HighSingleVol_sat : Saturate  UpperLimit=10  LowerLimit=0
  BMS2_HighSingleVolcv : DataTypeConversion
  BMS2_HighSingleVolinput1_Ad : Sum
  BMS2_HighSingleVolinput1_C : Constant  Value=256
  BMS2_HighSingleVolinput1_P : Product
  BMS2_LowSingleVol_Ad : Sum
  BMS2_LowSingleVol_Convert : DataTypeConversion  OutDataTypeStr=uint32
  BMS2_LowSingleVol_F : Gain
  BMS2_LowSingleVol_L : simulink/Logic and Bit Operations/Bitwise Operator  logicop=AND  UseBitMask=on  BitMask=65535  BitMaskRealWorld=Stored Integer
  BMS2_LowSingleVol_O : Constant  Value=0  OutDataTypeStr=single
  BMS2_LowSingleVol_S : ArithShift
  BMS2_LowSingleVol_Sub : Subsystem
  BMS2_LowSingleVol_sat : Saturate  UpperLimit=65535  LowerLimit=0
  BMS2_LowSingleVolcv : DataTypeConversion
  BMS2_LowSingleVolinput3_Ad : Sum
  BMS2_LowSingleVolinput3_C : Constant  Value=256
  BMS2_LowSingleVolinput3_P : Product
  Demux : Demux  Outputs=8
  BMS2_LowSingleVol_Out : Outport
  BMS2_HighSingleVol_Out : Outport  Port=2
  wires:
  BMS2_LowSingleVol_F/1 -> BMS2_LowSingleVol_Ad/1
  BMS2_LowSingleVol_O/1 -> BMS2_LowSingleVol_Ad/2
  BMS2_LowSingleVol_Ad/1 -> BMS2_LowSingleVol_sat/1
  BMS2_LowSingleVol_sat/1 -> BMS2_LowSingleVol_Out/1
  Demux/3 -> BMS2_LowSingleVolinput3_P/1
  BMS2_LowSingleVolinput3_C/1 -> BMS2_LowSingleVolinput3_P/2
  BMS2_LowSingleVolinput3_P/1 -> BMS2_LowSingleVolinput3_Ad/1
  Demux/4 -> BMS2_LowSingleVolinput3_Ad/2
  BMS2_LowSingleVolinput3_Ad/1 -> BMS2_LowSingleVol_Sub/1(In1)
  BMS2_LowSingleVol_Sub/1(Out1) -> BMS2_LowSingleVol_Convert/1
  BMS2_LowSingleVol_Convert/1 -> BMS2_LowSingleVol_L/1
  BMS2_LowSingleVol_L/1 -> BMS2_LowSingleVol_S/1
  BMS2_LowSingleVol_S/1 -> BMS2_LowSingleVolcv/1
  BMS2_LowSingleVolcv/1 -> BMS2_LowSingleVol_F/1
  BMS2_HighSingleVol_F/1 -> BMS2_HighSingleVol_Ad/1
  BMS2_HighSingleVol_O/1 -> BMS2_HighSingleVol_Ad/2
  BMS2_HighSingleVol_Ad/1 -> BMS2_HighSingleVol_sat/1
  BMS2_HighSingleVol_sat/1 -> BMS2_HighSingleVol_Out/1
  Demux/1 -> BMS2_HighSingleVolinput1_P/1
  BMS2_HighSingleVolinput1_C/1 -> BMS2_HighSingleVolinput1_P/2
  BMS2_HighSingleVolinput1_P/1 -> BMS2_HighSingleVolinput1_Ad/1
  Demux/2 -> BMS2_HighSingleVolinput1_Ad/2
  BMS2_HighSingleVolinput1_Ad/1 -> BMS2_HighSingleVol_Sub/1(In1)
  BMS2_HighSingleVol_Sub/1(Out1) -> BMS2_HighSingleVol_Convert/1
  BMS2_HighSingleVol_Convert/1 -> BMS2_HighSingleVol_L/1
  BMS2_HighSingleVol_L/1 -> BMS2_HighSingleVol_S/1
  BMS2_HighSingleVol_S/1 -> BMS2_HighSingleVolcv/1
  BMS2_HighSingleVolcv/1 -> BMS2_HighSingleVol_F/1
  input/1 -> Demux/1

== system six_plus_six_AcmsteeringV10_main/Data_input/BMS2_2/BMS2 ==
  input : Inport
  Enable : EnablePort
  BMS2_HighSingleVol_Ad : Sum
  BMS2_HighSingleVol_Convert : DataTypeConversion  OutDataTypeStr=uint32
  BMS2_HighSingleVol_F : Gain
  BMS2_HighSingleVol_L : simulink/Logic and Bit Operations/Bitwise Operator  logicop=AND  UseBitMask=on  BitMask=65535  BitMaskRealWorld=Stored Integer
  BMS2_HighSingleVol_O : Constant  Value=0  OutDataTypeStr=single
  BMS2_HighSingleVol_S : ArithShift
  BMS2_HighSingleVol_Sub : Subsystem
  BMS2_HighSingleVol_sat : Saturate  UpperLimit=10  LowerLimit=0
  BMS2_HighSingleVolcv : DataTypeConversion
  BMS2_HighSingleVolinput1_Ad : Sum
  BMS2_HighSingleVolinput1_C : Constant  Value=256
  BMS2_HighSingleVolinput1_P : Product
  BMS2_LowSingleVol_Ad : Sum
  BMS2_LowSingleVol_Convert : DataTypeConversion  OutDataTypeStr=uint32
  BMS2_LowSingleVol_F : Gain
  BMS2_LowSingleVol_L : simulink/Logic and Bit Operations/Bitwise Operator  logicop=AND  UseBitMask=on  BitMask=65535  BitMaskRealWorld=Stored Integer
  BMS2_LowSingleVol_O : Constant  Value=0  OutDataTypeStr=single
  BMS2_LowSingleVol_S : ArithShift
  BMS2_LowSingleVol_Sub : Subsystem
  BMS2_LowSingleVol_sat : Saturate  UpperLimit=65535  LowerLimit=0
  BMS2_LowSingleVolcv : DataTypeConversion
  BMS2_LowSingleVolinput3_Ad : Sum
  BMS2_LowSingleVolinput3_C : Constant  Value=256
  BMS2_LowSingleVolinput3_P : Product
  Demux : Demux  Outputs=8
  BMS2_LowSingleVol_Out : Outport
  BMS2_HighSingleVol_Out : Outport  Port=2
  wires:
  BMS2_LowSingleVol_F/1 -> BMS2_LowSingleVol_Ad/1
  BMS2_LowSingleVol_O/1 -> BMS2_LowSingleVol_Ad/2
  BMS2_LowSingleVol_Ad/1 -> BMS2_LowSingleVol_sat/1
  BMS2_LowSingleVol_sat/1 -> BMS2_LowSingleVol_Out/1
  Demux/3 -> BMS2_LowSingleVolinput3_P/1
  BMS2_LowSingleVolinput3_C/1 -> BMS2_LowSingleVolinput3_P/2
  BMS2_LowSingleVolinput3_P/1 -> BMS2_LowSingleVolinput3_Ad/1
  Demux/4 -> BMS2_LowSingleVolinput3_Ad/2
  BMS2_LowSingleVolinput3_Ad/1 -> BMS2_LowSingleVol_Sub/1(In1)
  BMS2_LowSingleVol_Sub/1(Out1) -> BMS2_LowSingleVol_Convert/1
  BMS2_LowSingleVol_Convert/1 -> BMS2_LowSingleVol_L/1
  BMS2_LowSingleVol_L/1 -> BMS2_LowSingleVol_S/1
  BMS2_LowSingleVol_S/1 -> BMS2_LowSingleVolcv/1
  BMS2_LowSingleVolcv/1 -> BMS2_LowSingleVol_F/1
  BMS2_HighSingleVol_F/1 -> BMS2_HighSingleVol_Ad/1
  BMS2_HighSingleVol_O/1 -> BMS2_HighSingleVol_Ad/2
  BMS2_HighSingleVol_Ad/1 -> BMS2_HighSingleVol_sat/1
  BMS2_HighSingleVol_sat/1 -> BMS2_HighSingleVol_Out/1
  Demux/1 -> BMS2_HighSingleVolinput1_P/1
  BMS2_HighSingleVolinput1_C/1 -> BMS2_HighSingleVolinput1_P/2
  BMS2_HighSingleVolinput1_P/1 -> BMS2_HighSingleVolinput1_Ad/1
  Demux/2 -> BMS2_HighSingleVolinput1_Ad/2
  BMS2_HighSingleVolinput1_Ad/1 -> BMS2_HighSingleVol_Sub/1(In1)
  BMS2_HighSingleVol_Sub/1(Out1) -> BMS2_HighSingleVol_Convert/1
  BMS2_HighSingleVol_Convert/1 -> BMS2_HighSingleVol_L/1
  BMS2_HighSingleVol_L/1 -> BMS2_HighSingleVol_S/1
  BMS2_HighSingleVol_S/1 -> BMS2_HighSingleVolcv/1
  BMS2_HighSingleVolcv/1 -> BMS2_HighSingleVol_F/1
  input/1 -> Demux/1
